simulink model "LKA"  (R2020b)
settings: Solver=FixedStepAuto  StartTime=0.0  StopTime=Inf  RelTol=1e-3
PostLoadFcn:
  | if any(exist('dsrtsu_mdlpostloadfcn', 'file') ~= 0), dsrtsu_mdlpostloadfcn('Execute', bdroot); end
InitFcn:
  | , if any(exist('dsmpb_private', 'file') ~= 0), dsmpb_private('dsmpb_mdlclblib', 'Init', bdroot); end,
PreSaveFcn:
  | , if any(exist('dsmpb_private', 'file') ~= 0), dsmpb_private('dsmpb_mdlclblib', 'PreSave', bdroot); end,
CloseFcn:
  | , if any(exist('dsmpb_private', 'file') ~= 0), dsmpb_private('dsmpb_mdlclblib', 'Close', bdroot); end,
settings Model: DataDictionary=HWA_DDs.sldd  RTICANMMDATA=struct('GeneralSetupData',struct('modelroot','F:\ADAS_Store\ADAS_Store\Adas\VSM\LSSState\LKA','generalsettings',struct('filesettings',struct('destfolder',struct('Name','RTICANMM_FILES','Check',1),'buildfolder',struct('Name','.','Check',1),'AbsDestfolder',struct('Name','F:\ADAS_Store\ADAS_Store\Adas\VSM\LSSState\LKA\RTICANMM_FILES'),'AbsBuildfolder',struct('Name','F:\ADAS_Store\ADAS_Store\Adas\VSM\LSSState\LKA'))),'options',struct('addpaths',1,'rmpaths',1,'addtrcexclusion',false,'cannavigator',struct('checkmonitoring',0),'show_usrtrc',0,'use_usrtrc',0),'advanced',struct('options',ones(1,100)),'MPSetup',{{}},'RTI',struct('Type','DSRT','Ver','4.2','Date','02-Nov-2019'),'modelname','LKA','block','LKA'))  DSRTSU_INTERNAL_RTIFPGA=150  Creator=GW00199575  LastModifiedBy=GW00199575
settings OptimizationCC: BlockReduction=off  ConditionallyExecuteInputs=off  OptimizeBlockIOStorage=off  BufferReuse=off
settings DebuggingCC: TasksWithSamePriorityMsg=none
settings HardwareCC: ProdBitPerPointer=32  ProdBitPerSizeT=32  ProdBitPerPtrDiffT=32  ProdLargestAtomicInteger=Integer  ProdWordSize=32  ProdHWDeviceType=Custom Processor->Custom
settings ModelReferenceCC: ModelReferenceNumInstancesAllowed=Single
settings SFSimCC: MATLABDynamicMemAlloc=off
settings RTWCC: Description=dSPACE Run-Time Target (for VEOS on Windows and ConfigurationDesk)  SystemTargetFile=dsrt.tlc  GenCodeOnly=on  MakeCommand=make_dsrt  TemplateMakefile=dsrt_default_tmf  RTWVerbose=off
settings CodeAppCC: MaxIdLength=128
settings STFCustomTargetCC: TargetLangStandard=C99 (ISO)  ParMdlRefBuildCompliant=on  ConcurrentExecutionCompliant=off  CPPClassGenCompliant=off  GRTInterface=off  SystemTargetFile=dsrt.tlc
settings GRTTargetCC: CompOptLevelCompliant=off  ConcurrentExecutionCompliant=off  CombineOutputUpdateFcns=off  MatFileLogging=off  CPPClassGenCompliant=off  UseToolchainInfoCompliant=off

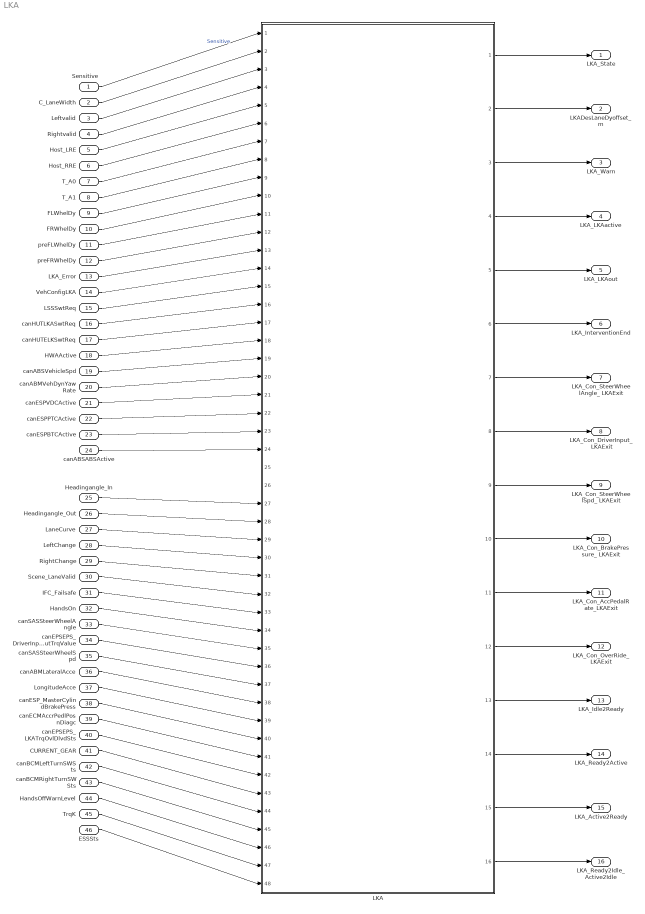
== system LKA ==
  Sensitive : Inport  OutDataTypeStr=uint8
  C_LaneWidth : Inport  Port=2  OutDataTypeStr=single
  Leftvalid : Inport  Port=3  OutDataTypeStr=boolean
  Rightvalid : Inport  Port=4  OutDataTypeStr=boolean
  Host_LRE : Inport  Port=5  OutDataTypeStr=boolean
  Host_RRE : Inport  Port=6  OutDataTypeStr=boolean
  T_A0 : Inport  Port=7  OutDataTypeStr=single
  T_A1 : Inport  Port=8  OutDataTypeStr=single
  FLWhelDy : Inport  Port=9  OutDataTypeStr=single
  FRWhelDy : Inport  Port=10  OutDataTypeStr=single
  preFLWhelDy : Inport  Port=11  OutDataTypeStr=single
  preFRWhelDy : Inport  Port=12  OutDataTypeStr=single
  LKA_Error : Inport  Port=13  OutDataTypeStr=boolean
  VehConfigLKA : Inport  Port=14  OutDataTypeStr=uint8
  LSSSwtReq : Inport  Port=15  OutDataTypeStr=boolean
  canHUTLKASwtReq : Inport  Port=16  OutDataTypeStr=boolean
  canHUTELKSwtReq : Inport  Port=17  OutDataTypeStr=boolean
  HWAActive : Inport  Port=18  OutDataTypeStr=boolean
  canABSVehicleSpd : Inport  Port=19  OutDataTypeStr=single
  canABMVehDynYawRate : Inport  Port=20  OutDataTypeStr=single
  canESPVDCActive : Inport  Port=21  OutDataTypeStr=boolean
  canESPPTCActive : Inport  Port=22  OutDataTypeStr=boolean
  canESPBTCActive : Inport  Port=23  OutDataTypeStr=boolean
  canABSABSActive : Inport  Port=24  OutDataTypeStr=boolean
  Headingangle_In : Inport  Port=25  OutDataTypeStr=boolean
  Headingangle_Out : Inport  Port=26  OutDataTypeStr=boolean
  LaneCurve : Inport  Port=27  OutDataTypeStr=single
  LeftChange : Inport  Port=28  OutDataTypeStr=boolean
  RightChange : Inport  Port=29  OutDataTypeStr=boolean
  Scene_LaneValid : Inport  Port=30  OutDataTypeStr=single
  IFC_Failsafe : Inport  Port=31  OutDataTypeStr=double
  HandsOn : Inport  Port=32  OutDataTypeStr=boolean
  canSASSteerWheelAngle : Inport  Port=33  OutDataTypeStr=single
  canEPSEPS_DriverInputTrqValue : Inport  Port=34  OutDataTypeStr=single
  canSASSteerWheelSpd : Inport  Port=35  OutDataTypeStr=single
  canABMLateralAcce : Inport  Port=36  OutDataTypeStr=single
  LongitudeAcce : Inport  Port=37  OutDataTypeStr=single
  canESP_MasterCylindBrakePress : Inport  Port=38  OutDataTypeStr=single
  canECMAccrPedlPosnDiagc : Inport  Port=39  OutDataTypeStr=single
  canEPSEPS_LKATrqOvlDlvdSts : Inport  Port=40  OutDataTypeStr=uint8
  CURRENT_GEAR : Inport  Port=41  OutDataTypeStr=uint8
  canBCMLeftTurnSWSts : Inport  Port=42  OutDataTypeStr=boolean
  canBCMRightTurnSWSts : Inport  Port=43  OutDataTypeStr=boolean
  HandsOffWarnLevel : Inport  Port=44  OutDataTypeStr=uint8
  TrqK : Inport  Port=45  OutDataTypeStr=single
  ESSSts : Inport  Port=46  OutDataTypeStr=uint8
  LKA : Subsystem  ReferencedSubsystem=PvtSubSys_VSM_LKA
  LKA_State : Outport
  LKADesLaneDyoffset_m : Outport  Port=2
  LKA_Warn : Outport  Port=3
  LKA_LKAactive : Outport  Port=4
  LKA_LKAout : Outport  Port=5
  LKA_InterventionEnd : Outport  Port=6
  LKA_Con_SteerWheelAngle_ LKAExit : Outport  Port=7
  LKA_Con_DriverInput_ LKAExit : Outport  Port=8
  LKA_Con_SteerWheelSpd_ LKAExit : Outport  Port=9
  LKA_Con_BrakePressure_ LKAExit : Outport  Port=10
  LKA_Con_AccPedalRate_LKAExit : Outport  Port=11
  LKA_Con_OverRide_ LKAExit : Outport  Port=12
  LKA_Idle2Ready : Outport  Port=13
  LKA_Ready2Active : Outport  Port=14
  LKA_Active2Ready : Outport  Port=15
  LKA_Ready2Idle_Active2Idle : Outport  Port=16
  wires:
  LKA/1 -> LKA_State/1
  LKA/2 -> LKADesLaneDyoffset_m/1
  LKA/3 -> LKA_Warn/1
  LKA/4 -> LKA_LKAactive/1
  LKA/5 -> LKA_LKAout/1
  LKA/6 -> LKA_InterventionEnd/1
  LKA/7 -> LKA_Con_SteerWheelAngle_ LKAExit/1
  LKA/8 -> LKA_Con_DriverInput_ LKAExit/1
  LKA/9 -> LKA_Con_SteerWheelSpd_ LKAExit/1
  LKA/10 -> LKA_Con_BrakePressure_ LKAExit/1
  LKA/11 -> LKA_Con_AccPedalRate_LKAExit/1
  LKA/12 -> LKA_Con_OverRide_ LKAExit/1
  LKA/13 -> LKA_Idle2Ready/1
  LKA/14 -> LKA_Ready2Active/1
  LKA/15 -> LKA_Active2Ready/1
  LKA/16 -> LKA_Ready2Idle_Active2Idle/1
  Sensitive/1 -> LKA/1  "Sensitive"
  C_LaneWidth/1 -> LKA/2
  Leftvalid/1 -> LKA/3
  Rightvalid/1 -> LKA/4
  Host_LRE/1 -> LKA/5
  Host_RRE/1 -> LKA/6
  T_A0/1 -> LKA/7
  T_A1/1 -> LKA/8
  FLWhelDy/1 -> LKA/9
  FRWhelDy/1 -> LKA/10
  preFLWhelDy/1 -> LKA/11
  preFRWhelDy/1 -> LKA/12
  LKA_Error/1 -> LKA/13
  VehConfigLKA/1 -> LKA/14
  LSSSwtReq/1 -> LKA/15
  canHUTLKASwtReq/1 -> LKA/16
  canHUTELKSwtReq/1 -> LKA/17
  HWAActive/1 -> LKA/18
  canABSVehicleSpd/1 -> LKA/19
  canABMVehDynYawRate/1 -> LKA/20
  canESPVDCActive/1 -> LKA/21
  canESPPTCActive/1 -> LKA/22
  canESPBTCActive/1 -> LKA/23
  canABSABSActive/1 -> LKA/24
  ESSSts/1 -> LKA/48
  TrqK/1 -> LKA/47
  HandsOn/1 -> LKA/34
  canSASSteerWheelAngle/1 -> LKA/35
  canEPSEPS_DriverInputTrqValue/1 -> LKA/36
  canSASSteerWheelSpd/1 -> LKA/37
  canABMLateralAcce/1 -> LKA/38
  LongitudeAcce/1 -> LKA/39
  canESP_MasterCylindBrakePress/1 -> LKA/40
  canECMAccrPedlPosnDiagc/1 -> LKA/41
  canEPSEPS_LKATrqOvlDlvdSts/1 -> LKA/42
  CURRENT_GEAR/1 -> LKA/43
  canBCMLeftTurnSWSts/1 -> LKA/44
  canBCMRightTurnSWSts/1 -> LKA/45
  HandsOffWarnLevel/1 -> LKA/46
  IFC_Failsafe/1 -> LKA/33
  Headingangle_In/1 -> LKA/27
  Headingangle_Out/1 -> LKA/28
  LaneCurve/1 -> LKA/29
  LeftChange/1 -> LKA/30
  RightChange/1 -> LKA/31
  Scene_LaneValid/1 -> LKA/32
